simulink model "Full_Car_Model"  (R2020a)
settings: Solver=ode4  StartTime=0  StopTime=3  FixedStep=0.001  RelTol=1e-3
undefined symbols (not defined in the file): a_CG, b_CG, Cs_FL, Cs_FR, Cs_RL, Cs_RR, g, Ip, Ir, Ks_FL, Ks_FR, Ks_RL, Ks_RR, Ms, mus1, mus2, mus3, mus4, tr
settings Model: Creator=anish  LastModifiedBy=anish
settings DataIOCC: ReturnWorkspaceOutputs=off
settings DebuggingCC: PregeneratedLibrarySubsystemCodeDiagnostic=none  ArithmeticOperatorsInVariantConditions=warning
settings SFSimCC: SimUseLocalCustomCode=off  CustomCodeUndefinedFunction=UseInterfaceOnly
settings RTWCC: RTWUseLocalCustomCode=off

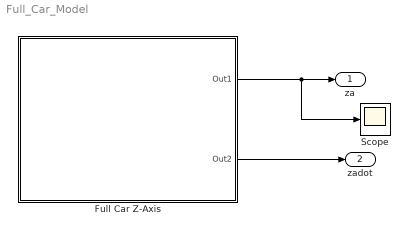
== system Full_Car_Model ==
  Full Car Z-Axis : Subsystem
  Scope : Scope
  za : Outport  VectorParamsAs1DForOutWhenUnconnected=off
  zadot : Outport  Port=2  VectorParamsAs1DForOutWhenUnconnected=off
  wires:
  Full Car Z-Axis/1(Out1) -> Scope/1, za/1
  Full Car Z-Axis/2(Out2) -> zadot/1

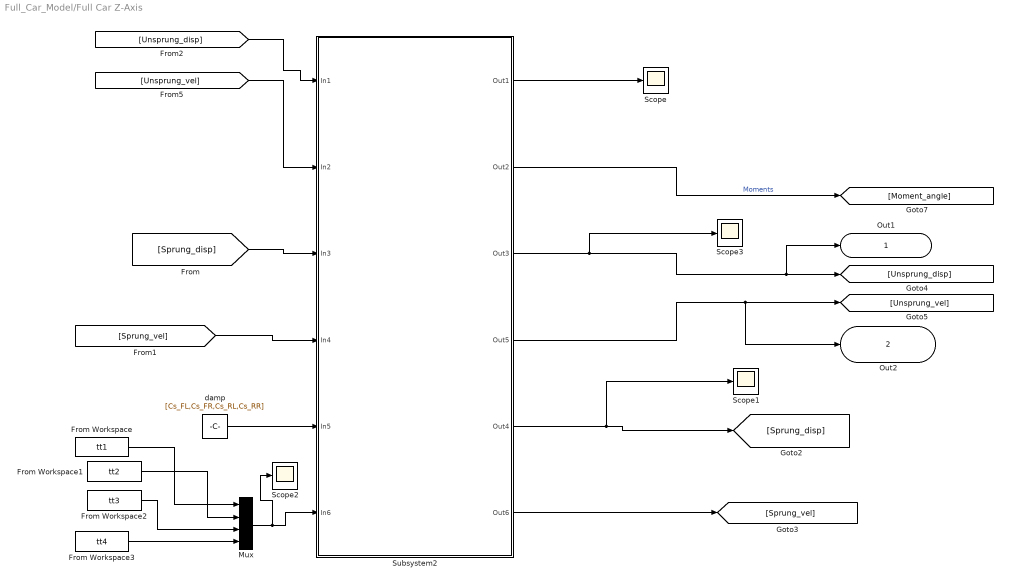
== system Full_Car_Model/Full Car Z-Axis ==
  From Workspace : FromWorkspace  VariableName=tt1  OutputAfterFinalValue=Setting to zero
  From Workspace1 : FromWorkspace  VariableName=tt2  OutputAfterFinalValue=Setting to zero
  From Workspace2 : FromWorkspace  VariableName=tt3  OutputAfterFinalValue=Setting to zero
  From Workspace3 : FromWorkspace  VariableName=tt4  OutputAfterFinalValue=Setting to zero
  Mux : Mux
  Scope{,1..3} (4 alike) : Scope
  Subsystem2 : Subsystem
  damp : Constant  Value=[Cs_FL,Cs_FR,Cs_RL,Cs_RR]
  Out1 : Outport  VectorParamsAs1DForOutWhenUnconnected=off
  Out2 : Outport  Port=2  VectorParamsAs1DForOutWhenUnconnected=off
  wires:
  [Unsprung_disp] -> Subsystem2/1(In1)
  [Unsprung_vel] -> Subsystem2/2(In2)
  damp/1 -> Subsystem2/5(In5)
  [Sprung_disp] -> Subsystem2/3(In3)
  [Sprung_vel] -> Subsystem2/4(In4)
  Subsystem2/3(Out3) -> Scope3/1, Out1/1, [Unsprung_disp]
  Subsystem2/4(Out5) -> Out2/1, [Unsprung_vel]
  Subsystem2/6(Out6) -> [Sprung_vel]
  Subsystem2/2(Out2) -> [Moment_angle]  "Moments"
  Subsystem2/1(Out1) -> Scope/1
  Mux/1 -> Scope2/1, Subsystem2/6(In6)
  From Workspace/1 -> Mux/1
  From Workspace1/1 -> Mux/2
  From Workspace2/1 -> Mux/3
  From Workspace3/1 -> Mux/4
  Subsystem2/5(Out4) -> Scope1/1, [Sprung_disp]

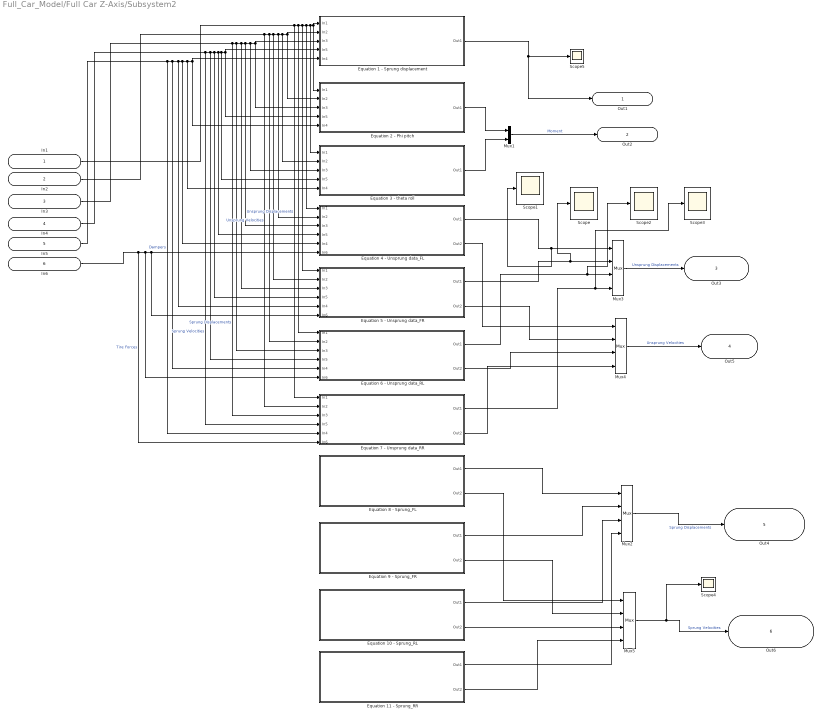
== system Full_Car_Model/Full Car Z-Axis/Subsystem2 ==
  In1 : Inport
  In2 : Inport  Port=2
  In3 : Inport  Port=3
  In4 : Inport  Port=4
  In5 : Inport  Port=5
  In6 : Inport  Port=6
  Equation 1 - Sprung displacement : Subsystem
  Equation 10 - Sprung_RL : Subsystem
  Equation 11 - Sprung_RR : Subsystem
  Equation 2 - Phi pitch : Subsystem
  Equation 3 - theta roll : Subsystem
  Equation 4 - Unsprung data_FL : Subsystem
  Equation 5 - Unsprung data_FR : Subsystem
  Equation 6 - Unsprung data_RL : Subsystem
  Equation 7 - Unsprung data_RR : Subsystem
  Equation 8 - Sprung_FL : Subsystem
  Equation 9 - Sprung_FR : Subsystem
  Mux1 : Mux  Inputs=2
  Mux{2..5} (4 alike) : Mux
  Scope{,1..5} (6 alike) : Scope
  Out1 : Outport  VectorParamsAs1DForOutWhenUnconnected=off
  Out2 : Outport  Port=2  VectorParamsAs1DForOutWhenUnconnected=off
  Out3 : Outport  Port=3  VectorParamsAs1DForOutWhenUnconnected=off
  Out5 : Outport  Port=4  VectorParamsAs1DForOutWhenUnconnected=off
  Out4 : Outport  Port=5  VectorParamsAs1DForOutWhenUnconnected=off
  Out6 : Outport  Port=6  VectorParamsAs1DForOutWhenUnconnected=off
  wires:
  Mux1/1 -> Out2/1  "Moment"
  Equation 2 - Phi pitch/1(Out1) -> Mux1/1
  Equation 3 - theta roll/1(Out1) -> Mux1/2
  In1/1 -> Equation 7 - Unsprung data_RR/1(In1), Equation 6 - Unsprung data_RL/1(In1), Equation 5 - Unsprung data_FR/1(In1), Equation 4 - Unsprung data_FL/1(In1), Equation 3 - theta roll/1(In1), Equation 2 - Phi pitch/1(In1), Equation 1 - Sprung displacement/1(In1)  "Unsprung Displacements"
  In2/1 -> Equation 7 - Unsprung data_RR/2(In2), Equation 6 - Unsprung data_RL/2(In2), Equation 5 - Unsprung data_FR/2(In2), Equation 4 - Unsprung data_FL/2(In2), Equation 3 - theta roll/2(In2), Equation 2 - Phi pitch/2(In2), Equation 1 - Sprung displacement/2(In2)  "Unsprung Velocities"
  In3/1 -> Equation 7 - Unsprung data_RR/3(In3), Equation 6 - Unsprung data_RL/3(In3), Equation 5 - Unsprung data_FR/3(In3), Equation 4 - Unsprung data_FL/3(In3), Equation 3 - theta roll/3(In3), Equation 2 - Phi pitch/3(In3), Equation 1 - Sprung displacement/3(In3)  "Sprung Displacements"
  In4/1 -> Equation 7 - Unsprung data_RR/4(In5), Equation 6 - Unsprung data_RL/4(In5), Equation 5 - Unsprung data_FR/4(In5), Equation 4 - Unsprung data_FL/4(In5), Equation 3 - theta roll/4(In5), Equation 2 - Phi pitch/4(In5), Equation 1 - Sprung displacement/4(In5)  "Sprung Velocities"
  In5/1 -> Equation 7 - Unsprung data_RR/5(In4), Equation 6 - Unsprung data_RL/5(In4), Equation 5 - Unsprung data_FR/5(In4), Equation 4 - Unsprung data_FL/5(In4), Equation 3 - theta roll/5(In4), Equation 2 - Phi pitch/5(In4), Equation 1 - Sprung displacement/5(In4)  "Dampers"
  In6/1 -> Equation 7 - Unsprung data_RR/6(In6), Equation 6 - Unsprung data_RL/6(In6), Equation 5 - Unsprung data_FR/6(In6), Equation 4 - Unsprung data_FL/6(In6)  "Tire Forces"
  Equation 1 - Sprung displacement/1(Out1) -> Out1/1, Scope5/1
  Mux3/1 -> Out3/1  "Unsprung Displacements"
  Mux4/1 -> Out5/1  "Unsprung Velocities"
  Equation 4 - Unsprung data_FL/1(Out1) -> Scope1/1, Mux3/1
  Equation 5 - Unsprung data_FR/1(Out1) -> Scope/1, Mux3/2
  Equation 6 - Unsprung data_RL/1(Out1) -> Scope2/1, Mux3/3
  Equation 7 - Unsprung data_RR/1(Out1) -> Scope3/1, Mux3/4
  Equation 4 - Unsprung data_FL/2(Out2) -> Mux4/1
  Equation 5 - Unsprung data_FR/2(Out2) -> Mux4/2
  Equation 6 - Unsprung data_RL/2(Out2) -> Mux4/3
  Equation 7 - Unsprung data_RR/2(Out2) -> Mux4/4
  Mux2/1 -> Out4/1  "Sprung Displacements"
  Mux5/1 -> Scope4/1, Out6/1  "Sprung Velocities"
  Equation 8 - Sprung_FL/1(Out1) -> Mux2/1
  Equation 9 - Sprung_FR/1(Out1) -> Mux2/2
  Equation 10 - Sprung_RL/1(Out1) -> Mux2/3
  Equation 11 - Sprung_RR/1(Out1) -> Mux2/4
  Equation 8 - Sprung_FL/2(Out2) -> Mux5/1
  Equation 9 - Sprung_FR/2(Out2) -> Mux5/2
  Equation 10 - Sprung_RL/2(Out2) -> Mux5/3
  Equation 11 - Sprung_RR/2(Out2) -> Mux5/4

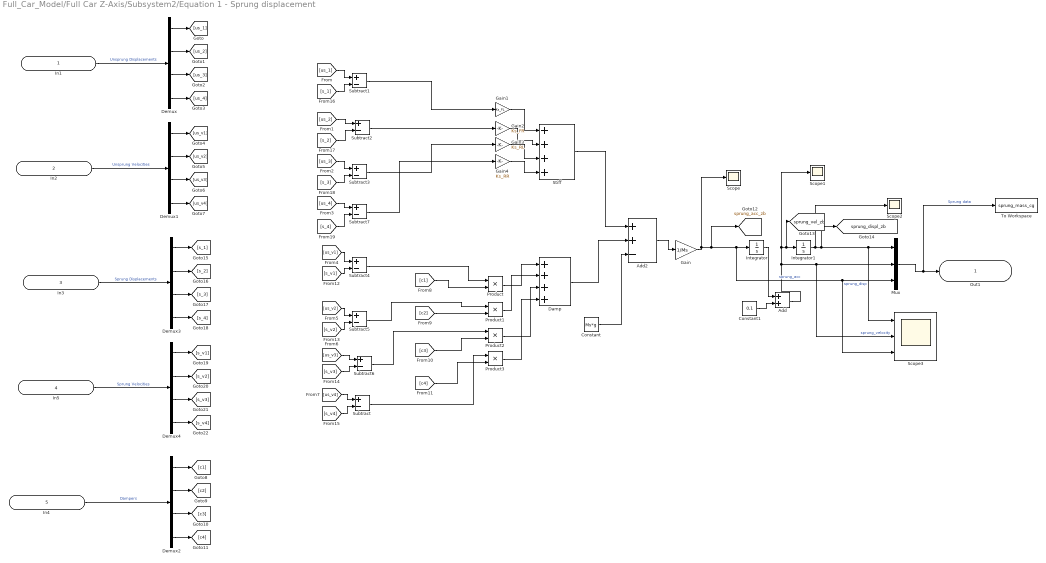
== system Full_Car_Model/Full Car Z-Axis/Subsystem2/Equation 1 - Sprung displacement ==
  In1 : Inport
  In2 : Inport  Port=2
  In3 : Inport  Port=3
  In5 : Inport  Port=4
  In4 : Inport  Port=5
  Add : Sum
  Add2 : Sum  Inputs=++-
  Constant : Constant  Value=Ms*g
  Constant1 : Constant  Value=0.1
  Damp : Sum  Inputs=++++
  Demux{,1..4} (5 alike) : Demux
  Gain : Gain  Gain=1/Ms
  Gain1 : Gain  Gain=Ks_FL
  Gain2 : Gain  Gain=Ks_FR
  Gain3 : Gain  Gain=Ks_RL
  Gain4 : Gain  Gain=Ks_RR
  Integrator : Integrator
  Integrator1 : Integrator  InitialCondition=-0.0177
  Mux : Mux  Inputs=3
  Product{,1..3} (4 alike) : Product
  Scope : Scope
  Scope1 : Scope
  Scope2 : Scope
  Scope3 : Scope  NumInputPorts=3
  Stiff : Sum  Inputs=++++
  Subtract{,1..7} (8 alike) : Sum  Inputs=+-
  To Workspace : ToWorkspace  VariableName=sprung_mass_cg  SampleTime=-1
      settings: Save2DSignal=2-D array (concatenate along first dimension)
  Out1 : Outport  VectorParamsAs1DForOutWhenUnconnected=off
  tag scope: sprung_acc_zb=global, sprung_displ_zb=global, sprung_vel_zb=global
  wires:
  In1/1 -> Demux/1  "Unsprung Displacements"
  Add2/1 -> Gain/1
  Damp/1 -> Add2/2
  Constant/1 -> Add2/3
  Gain/1 -> Scope/1, [sprung_acc_zb], Scope3/3, Mux/3, Integrator/1  "sprung_acc"
  Mux/1 -> To Workspace/1, Out1/1  "Sprung data"
  Demux/1 -> [us_1]
  Demux/2 -> [us_2]
  Demux/3 -> [us_3]
  Demux/4 -> [us_4]
  In2/1 -> Demux1/1  "Unsprung Velocities"
  Demux1/1 -> [us_v1]
  Demux1/4 -> [us_v4]
  Demux1/2 -> [us_v2]
  Demux1/3 -> [us_v3]
  In4/1 -> Demux2/1  "Dampers"
  Demux2/3 -> [c3]
  Demux2/2 -> [c2]
  Demux2/4 -> [c4]
  Demux2/1 -> [c1]
  Integrator1/1 -> Scope2/1, [sprung_displ_zb], Scope3/1, Mux/1  "sprung_disp"
  Gain1/1 -> Stiff/1
  Gain2/1 -> Stiff/2
  Gain3/1 -> Stiff/3
  Gain4/1 -> Stiff/4
  [c1] -> Product/2
  [c4] -> Product3/2
  [c3] -> Product2/2
  [c2] -> Product1/2
  Product/1 -> Damp/1
  Product1/1 -> Damp/2
  Product2/1 -> Damp/3
  Product3/1 -> Damp/4
  Demux4/4 -> [s_v4]
  Demux3/2 -> [s_2]
  Demux4/1 -> [s_v1]
  Demux3/4 -> [s_4]
  Demux3/3 -> [s_3]
  Demux3/1 -> [s_1]
  Demux4/2 -> [s_v2]
  Demux4/3 -> [s_v3]
  In5/1 -> Demux4/1  "Sprung Velocities"
  In3/1 -> Demux3/1  "Sprung Displacements"
  [us_v1] -> Subtract4/1
  [s_v1] -> Subtract4/2
  [us_v2] -> Subtract5/1
  [s_v2] -> Subtract5/2
  [us_v3] -> Subtract6/1
  [s_v3] -> Subtract6/2
  [us_v4] -> Subtract/1
  [s_v4] -> Subtract/2
  Subtract4/1 -> Product/1
  Subtract5/1 -> Product1/1
  Subtract6/1 -> Product2/1
  Subtract/1 -> Product3/1
  [us_1] -> Subtract1/1
  [s_1] -> Subtract1/2
  [us_2] -> Subtract2/1
  [s_2] -> Subtract2/2
  [us_3] -> Subtract3/1
  [s_3] -> Subtract3/2
  [us_4] -> Subtract7/1
  [s_4] -> Subtract7/2
  Stiff/1 -> Add2/1
  Subtract1/1 -> Gain1/1
  Subtract2/1 -> Gain2/1
  Subtract3/1 -> Gain3/1
  Subtract7/1 -> Gain4/1
  Constant1/1 -> Add/2
  Integrator/1 -> Add/1
  Add/1 -> Scope3/2, Mux/2, Scope1/1, [sprung_vel_zb], Integrator1/1  "sprung_velocity"

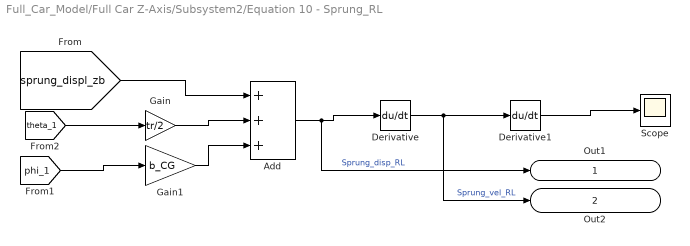
== system Full_Car_Model/Full Car Z-Axis/Subsystem2/Equation 10 - Sprung_RL ==
  Add : Sum  Inputs=+++
  Derivative : Derivative
  Derivative1 : Derivative
  Gain : Gain  Gain=tr/2
  Gain1 : Gain  Gain=b_CG
  Scope : Scope
  Out1 : Outport  VectorParamsAs1DForOutWhenUnconnected=off
  Out2 : Outport  Port=2  VectorParamsAs1DForOutWhenUnconnected=off
  wires:
  [sprung_displ_zb] -> Add/1
  Gain/1 -> Add/2
  Gain1/1 -> Add/3
  [phi_1] -> Gain1/1
  [theta_1] -> Gain/1
  Add/1 -> Out1/1, Derivative/1  "Sprung_disp_RL"
  Derivative/1 -> Out2/1, Derivative1/1  "Sprung_vel_RL"
  Derivative1/1 -> Scope/1

== system Full_Car_Model/Full Car Z-Axis/Subsystem2/Equation 11 - Sprung_RR ==
  Add : Sum  Inputs=+-+
  Derivative : Derivative
  Derivative1 : Derivative
  Gain : Gain  Gain=tr/2
  Gain1 : Gain  Gain=b_CG
  Scope : Scope
  Out1 : Outport  VectorParamsAs1DForOutWhenUnconnected=off
  Out2 : Outport  Port=2  VectorParamsAs1DForOutWhenUnconnected=off
  wires:
  [sprung_displ_zb] -> Add/1
  Gain/1 -> Add/2
  Gain1/1 -> Add/3
  [phi_1] -> Gain1/1
  [theta_1] -> Gain/1
  Add/1 -> Out1/1, Derivative/1  "Sprung_disp_RR"
  Derivative/1 -> Out2/1, Derivative1/1  "Sprung_vel_RR"
  Derivative1/1 -> Scope/1

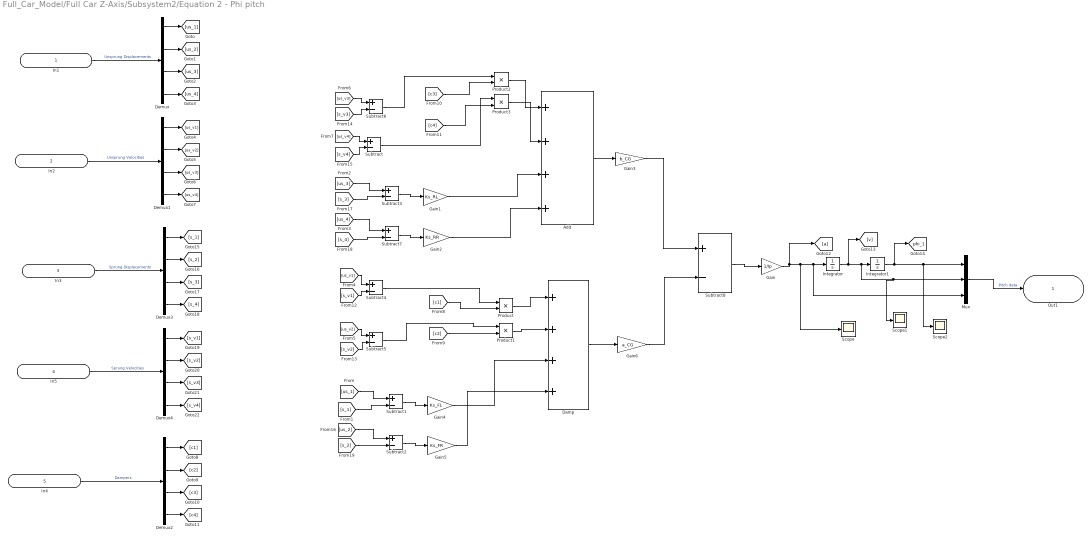
== system Full_Car_Model/Full Car Z-Axis/Subsystem2/Equation 2 - Phi pitch ==
  In1 : Inport
  In2 : Inport  Port=2
  In3 : Inport  Port=3
  In5 : Inport  Port=4
  In4 : Inport  Port=5
  Add : Sum  Inputs=++++
  Damp : Sum  Inputs=++++
  Demux{,1..4} (5 alike) : Demux
  Gain : Gain  Gain=1/Ip
  Gain1 : Gain  Gain=Ks_RL
  Gain2 : Gain  Gain=Ks_RR
  Gain3 : Gain  Gain=b_CG
  Gain4 : Gain  Gain=Ks_FL
  Gain5 : Gain  Gain=Ks_FR
  Gain6 : Gain  Gain=a_CG
  Integrator : Integrator  UpperSaturationLimit=0.00001  LowerSaturationLimit=-0.00001
  Integrator1 : Integrator  UpperSaturationLimit=0.00001  LowerSaturationLimit=-0.00001
  Mux : Mux  Inputs=3
  Product{,1..3} (4 alike) : Product
  Scope : Scope
  Scope1 : Scope
  Scope2 : Scope
  Subtract{,1..8} (9 alike) : Sum  Inputs=+-
  Out1 : Outport  VectorParamsAs1DForOutWhenUnconnected=off
  tag scope: phi_1=global
  wires:
  In1/1 -> Demux/1  "Unsprung Displacements"
  Subtract8/1 -> Gain/1
  Gain/1 -> [a], Scope/1, Mux/3, Integrator/1
  Integrator/1 -> [v], Scope1/1, Mux/2, Integrator1/1
  Mux/1 -> Out1/1  "Pitch data"
  Demux/1 -> [us_1]
  Demux/2 -> [us_2]
  Demux/3 -> [us_3]
  Demux/4 -> [us_4]
  In2/1 -> Demux1/1  "Unsprung Velocities"
  Demux1/1 -> [us_v1]
  Demux1/4 -> [us_v4]
  Demux1/2 -> [us_v2]
  Demux1/3 -> [us_v3]
  In4/1 -> Demux2/1  "Dampers"
  Demux2/3 -> [c3]
  Demux2/2 -> [c2]
  Demux2/4 -> [c4]
  Demux2/1 -> [c1]
  Integrator1/1 -> [phi_1], Scope2/1, Mux/1
  [c1] -> Product/2
  [c2] -> Product1/2
  Product/1 -> Damp/1
  Product1/1 -> Damp/2
  Demux4/4 -> [s_v4]
  Demux3/2 -> [s_2]
  Demux4/1 -> [s_v1]
  Demux3/4 -> [s_4]
  Demux3/3 -> [s_3]
  Demux3/1 -> [s_1]
  Demux4/2 -> [s_v2]
  Demux4/3 -> [s_v3]
  In5/1 -> Demux4/1  "Sprung Velocities"
  In3/1 -> Demux3/1  "Sprung Displacements"
  [us_v1] -> Subtract4/1
  [s_v1] -> Subtract4/2
  [us_v2] -> Subtract5/1
  [s_v2] -> Subtract5/2
  Subtract4/1 -> Product/1
  Subtract5/1 -> Product1/1
  [us_2] -> Subtract2/1
  [s_1] -> Subtract1/2
  Subtract2/1 -> Gain5/1
  Subtract1/1 -> Gain4/1
  [us_1] -> Subtract1/1
  [s_2] -> Subtract2/2
  Gain4/1 -> Damp/3
  Gain5/1 -> Damp/4
  Damp/1 -> Gain6/1
  Product2/1 -> Add/1
  Subtract3/1 -> Gain1/1
  Gain1/1 -> Add/3
  [c3] -> Product2/2
  [c4] -> Product3/2
  [s_v3] -> Subtract6/2
  [us_v4] -> Subtract/1
  Subtract6/1 -> Product2/1
  Subtract/1 -> Product3/1
  [s_3] -> Subtract3/2
  Gain2/1 -> Add/4
  [s_v4] -> Subtract/2
  [us_v3] -> Subtract6/1
  Subtract7/1 -> Gain2/1
  Product3/1 -> Add/2
  [us_3] -> Subtract3/1
  [s_4] -> Subtract7/2
  Add/1 -> Gain3/1
  [us_4] -> Subtract7/1
  Gain3/1 -> Subtract8/1
  Gain6/1 -> Subtract8/2

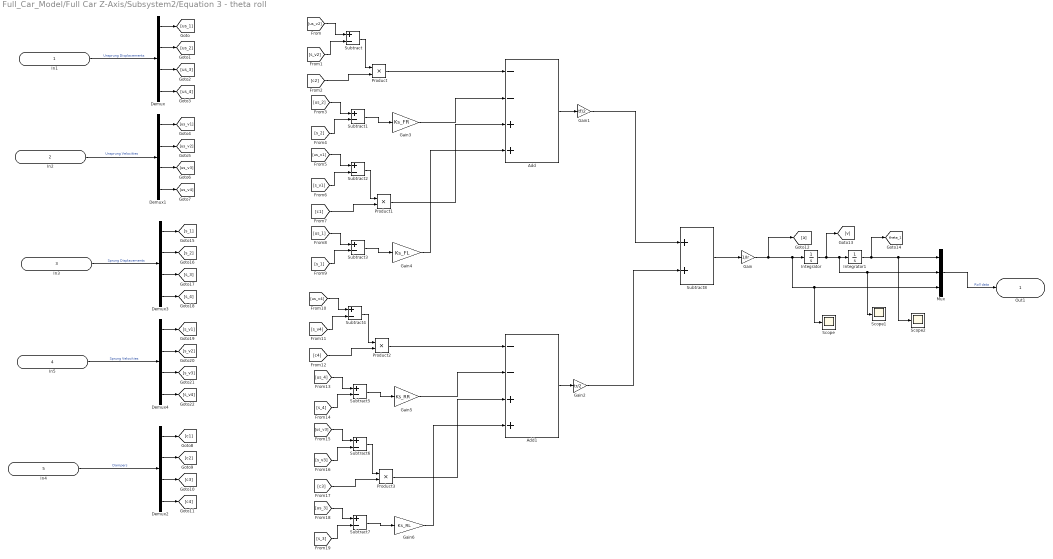
== system Full_Car_Model/Full Car Z-Axis/Subsystem2/Equation 3 - theta roll ==
  In1 : Inport
  In2 : Inport  Port=2
  In3 : Inport  Port=3
  In5 : Inport  Port=4
  In4 : Inport  Port=5
  Add : Sum  Inputs=--++
  Add1 : Sum  Inputs=--++
  Demux{,1..4} (5 alike) : Demux
  Gain : Gain  Gain=1/Ir
  Gain1 : Gain  Gain=tf/2
  Gain2 : Gain  Gain=tr/2
  Gain3 : Gain  Gain=Ks_FR
  Gain4 : Gain  Gain=Ks_FL
  Gain5 : Gain  Gain=Ks_RR
  Gain6 : Gain  Gain=Ks_RL
  Integrator : Integrator  UpperSaturationLimit=0.00001  LowerSaturationLimit=-0.00001
  Integrator1 : Integrator  UpperSaturationLimit=0.00001  LowerSaturationLimit=-0.00001
  Mux : Mux  Inputs=3
  Product{,1..3} (4 alike) : Product
  Scope : Scope
  Scope1 : Scope
  Scope2 : Scope
  Subtract{,1..7} (8 alike) : Sum  Inputs=+-
  Subtract8 : Sum
  Out1 : Outport  VectorParamsAs1DForOutWhenUnconnected=off
  tag scope: theta_1=global
  wires:
  In1/1 -> Demux/1  "Unsprung Displacements"
  Subtract8/1 -> Gain/1
  Integrator/1 -> [v], Scope1/1, Mux/2, Integrator1/1
  Mux/1 -> Out1/1  "Roll data"
  Demux/1 -> [us_1]
  Demux/2 -> [us_2]
  Demux/3 -> [us_3]
  Demux/4 -> [us_4]
  In2/1 -> Demux1/1  "Unsprung Velocities"
  Demux1/1 -> [us_v1]
  Demux1/4 -> [us_v4]
  Demux1/2 -> [us_v2]
  Demux1/3 -> [us_v3]
  In4/1 -> Demux2/1  "Dampers"
  Demux2/3 -> [c3]
  Demux2/2 -> [c2]
  Demux2/4 -> [c4]
  Demux2/1 -> [c1]
  Integrator1/1 -> [theta_1], Scope2/1, Mux/1
  Demux4/4 -> [s_v4]
  Demux3/2 -> [s_2]
  Demux4/1 -> [s_v1]
  Demux3/4 -> [s_4]
  Demux3/3 -> [s_3]
  Demux3/1 -> [s_1]
  Demux4/2 -> [s_v2]
  Demux4/3 -> [s_v3]
  In5/1 -> Demux4/1  "Sprung Velocities"
  In3/1 -> Demux3/1  "Sprung Displacements"
  Add/1 -> Gain1/1
  Add1/1 -> Gain2/1
  [us_v2] -> Subtract/1
  [s_v2] -> Subtract/2
  Subtract/1 -> Product/1
  [c2] -> Product/2
  Product/1 -> Add/1
  [s_2] -> Subtract1/2
  [us_2] -> Subtract1/1
  Subtract1/1 -> Gain3/1
  Gain3/1 -> Add/2
  [c1] -> Product1/2
  [s_v1] -> Subtract2/2
  Subtract2/1 -> Product1/1
  [us_v1] -> Subtract2/1
  Product1/1 -> Add/3
  [s_1] -> Subtract3/2
  [us_1] -> Subtract3/1
  Subtract3/1 -> Gain4/1
  Gain4/1 -> Add/4
  [us_v3] -> Subtract6/1
  [c3] -> Product3/2
  [s_v3] -> Subtract6/2
  [s_4] -> Subtract5/2
  [us_4] -> Subtract5/1
  [s_3] -> Subtract7/2
  Subtract5/1 -> Gain5/1
  Product3/1 -> Add1/3
  Product2/1 -> Add1/1
  Gain5/1 -> Add1/2
  Subtract6/1 -> Product3/1
  Gain6/1 -> Add1/4
  [us_3] -> Subtract7/1
  [c4] -> Product2/2
  [s_v4] -> Subtract4/2
  Subtract7/1 -> Gain6/1
  Subtract4/1 -> Product2/1
  [us_v4] -> Subtract4/1
  Gain1/1 -> Subtract8/1
  Gain2/1 -> Subtract8/2
  Gain/1 -> [a], Scope/1, Mux/3, Integrator/1

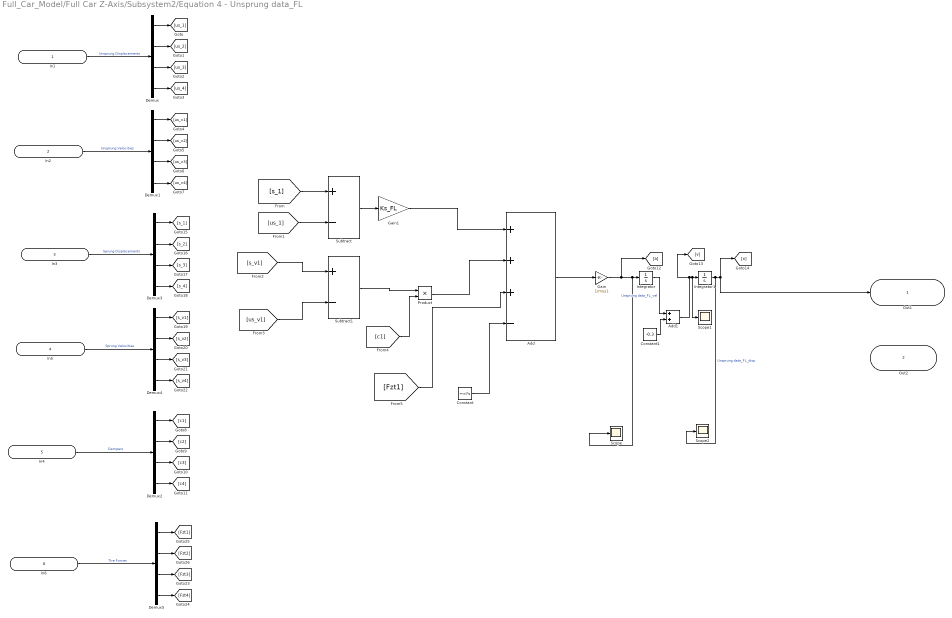
== system Full_Car_Model/Full Car Z-Axis/Subsystem2/Equation 4 - Unsprung data_FL ==
  In1 : Inport
  In2 : Inport  Port=2
  In3 : Inport  Port=3
  In5 : Inport  Port=4
  In4 : Inport  Port=5
  In6 : Inport  Port=6
  Add : Sum  Inputs=+++-
  Add1 : Sum
  Constant : Constant  Value=mus1*g
  Constant1 : Constant  Value=-0.3
  Demux{,1..5} (6 alike) : Demux
  Gain : Gain  Gain=1/mus1
  Gain1 : Gain  Gain=Ks_FL
  Integrator : Integrator
  Integrator1 : Integrator  InitialCondition=-0.0177
  Product : Product
  Scope : Scope
  Scope1 : Scope
  Scope2 : Scope
  Subtract : Sum  Inputs=+-
  Subtract1 : Sum  Inputs=+-
  Out1 : Outport  VectorParamsAs1DForOutWhenUnconnected=off
  Out2 : Outport  Port=2  VectorParamsAs1DForOutWhenUnconnected=off
  wires:
  In1/1 -> Demux/1  "Unsprung Displacements"
  Add/1 -> Gain/1
  Integrator1/1 -> Scope2/1, Out1/1, [x]  "Unsprung data_FL_disp"
  Demux/1 -> [us_1]
  Demux/2 -> [us_2]
  Demux/3 -> [us_3]
  Demux/4 -> [us_4]
  In2/1 -> Demux1/1  "Unsprung Velocities"
  Demux1/1 -> [us_v1]
  Demux1/4 -> [us_v4]
  Demux1/2 -> [us_v2]
  Demux1/3 -> [us_v3]
  In4/1 -> Demux2/1  "Dampers"
  Demux2/3 -> [c3]
  Demux2/2 -> [c2]
  Demux2/4 -> [c4]
  Demux2/1 -> [c1]
  Demux4/4 -> [s_v4]
  Demux3/2 -> [s_2]
  Demux4/1 -> [s_v1]
  Demux3/4 -> [s_4]
  Demux3/3 -> [s_3]
  Demux3/1 -> [s_1]
  Demux4/2 -> [s_v2]
  Demux4/3 -> [s_v3]
  In5/1 -> Demux4/1  "Sprung Velocities"
  In3/1 -> Demux3/1  "Sprung Displacements"
  In6/1 -> Demux5/1  "Tire Forces"
  Demux5/2 -> [Fzt2]
  Demux5/3 -> [Fzt3]
  Demux5/1 -> [Fzt1]
  Demux5/4 -> [Fzt4]
  [us_1] -> Subtract/2
  [s_1] -> Subtract/1
  Subtract/1 -> Gain1/1
  [s_v1] -> Subtract1/1
  [us_v1] -> Subtract1/2
  Subtract1/1 -> Product/1
  [c1] -> Product/2
  Gain1/1 -> Add/1
  Product/1 -> Add/2
  [Fzt1] -> Add/3
  Constant/1 -> Add/4
  Gain/1 -> [a], Scope/1, Integrator/1
  Constant1/1 -> Add1/2
  Integrator/1 -> Add1/1  "Unsprung data_FL_vel"
  Add1/1 -> Scope1/1, Integrator1/1, [v]

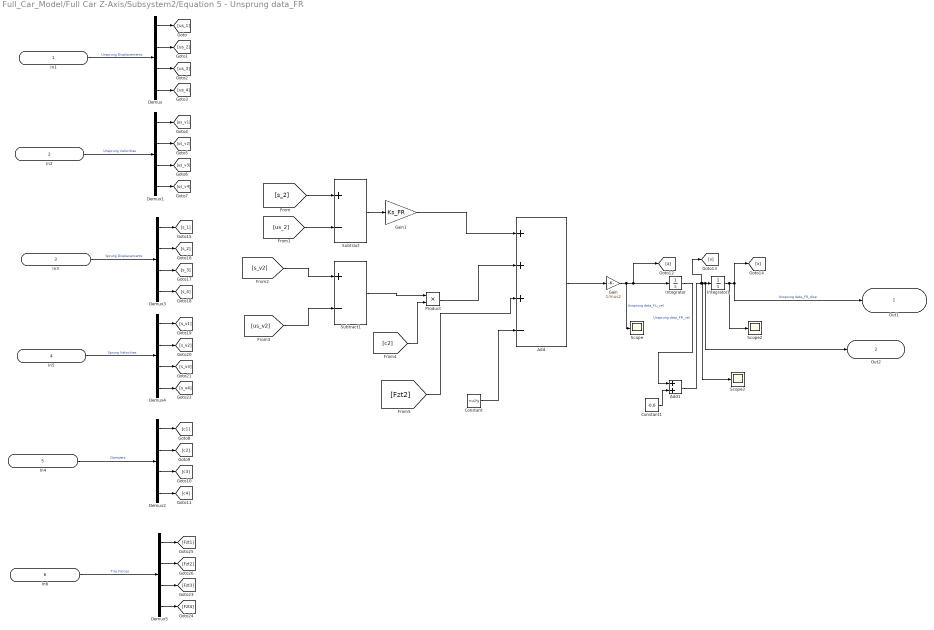
== system Full_Car_Model/Full Car Z-Axis/Subsystem2/Equation 5 - Unsprung data_FR ==
  In1 : Inport
  In2 : Inport  Port=2
  In3 : Inport  Port=3
  In5 : Inport  Port=4
  In4 : Inport  Port=5
  In6 : Inport  Port=6
  Add : Sum  Inputs=+++-
  Add1 : Sum
  Constant : Constant  Value=mus2*g
  Constant1 : Constant  Value=-0.6
  Demux{,1..5} (6 alike) : Demux
  Gain : Gain  Gain=1/mus2
  Gain1 : Gain  Gain=Ks_FR
  Integrator : Integrator
  Integrator1 : Integrator  InitialCondition=-0.0177
  Product : Product
  Scope : Scope
  Scope2 : Scope
  Scope3 : Scope
  Subtract : Sum  Inputs=+-
  Subtract1 : Sum  Inputs=+-
  Out1 : Outport  VectorParamsAs1DForOutWhenUnconnected=off
  Out2 : Outport  Port=2  VectorParamsAs1DForOutWhenUnconnected=off
  wires:
  In1/1 -> Demux/1  "Unsprung Displacements"
  Add/1 -> Gain/1
  Integrator1/1 -> Scope2/1, Out1/1, [x]  "Unsprung data_FR_disp"
  Demux/1 -> [us_1]
  Demux/2 -> [us_2]
  Demux/3 -> [us_3]
  Demux/4 -> [us_4]
  In2/1 -> Demux1/1  "Unsprung Velocities"
  Demux1/1 -> [us_v1]
  Demux1/4 -> [us_v4]
  Demux1/2 -> [us_v2]
  Demux1/3 -> [us_v3]
  In4/1 -> Demux2/1  "Dampers"
  Demux2/3 -> [c3]
  Demux2/2 -> [c2]
  Demux2/4 -> [c4]
  Demux2/1 -> [c1]
  Demux4/4 -> [s_v4]
  Demux3/2 -> [s_2]
  Demux4/1 -> [s_v1]
  Demux3/4 -> [s_4]
  Demux3/3 -> [s_3]
  Demux3/1 -> [s_1]
  Demux4/2 -> [s_v2]
  Demux4/3 -> [s_v3]
  In5/1 -> Demux4/1  "Sprung Velocities"
  In3/1 -> Demux3/1  "Sprung Displacements"
  In6/1 -> Demux5/1  "Tire Forces"
  Demux5/2 -> [Fzt2]
  Demux5/3 -> [Fzt3]
  Demux5/1 -> [Fzt1]
  Demux5/4 -> [Fzt4]
  [us_2] -> Subtract/2
  [s_2] -> Subtract/1
  Subtract/1 -> Gain1/1
  [s_v2] -> Subtract1/1
  [us_v2] -> Subtract1/2
  Subtract1/1 -> Product/1
  [c2] -> Product/2
  Gain1/1 -> Add/1
  Product/1 -> Add/2
  [Fzt2] -> Add/3
  Constant/1 -> Add/4
  Constant1/1 -> Add1/2
  Gain/1 -> Scope/1, [a], Integrator/1  "Unsprung data_FL_vel"
  Integrator/1 -> Add1/1  "Unsprung data_FR_vel"
  Add1/1 -> [v], Scope3/1, Out2/1, Integrator1/1

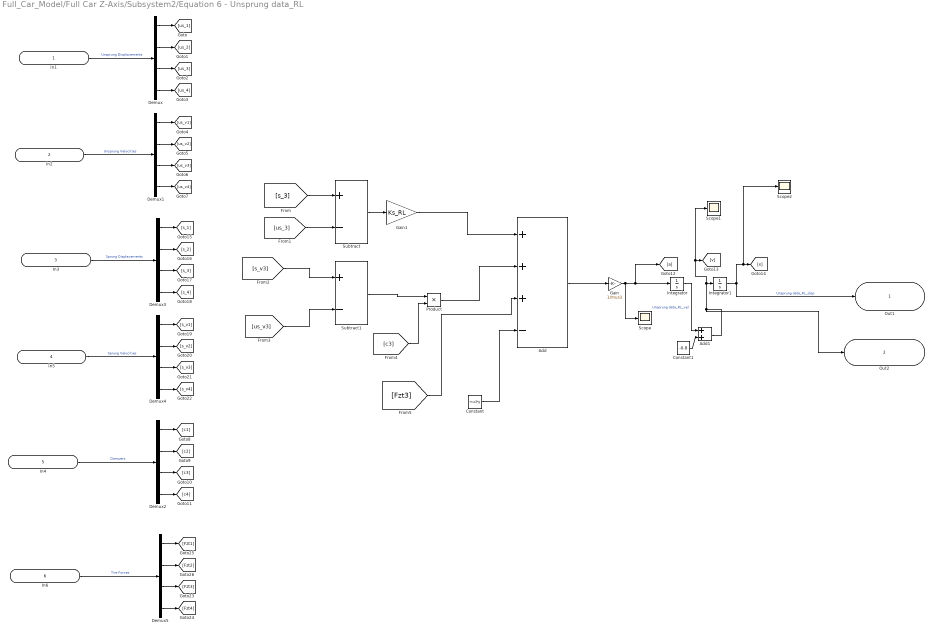
== system Full_Car_Model/Full Car Z-Axis/Subsystem2/Equation 6 - Unsprung data_RL ==
  In1 : Inport
  In2 : Inport  Port=2
  In3 : Inport  Port=3
  In5 : Inport  Port=4
  In4 : Inport  Port=5
  In6 : Inport  Port=6
  Add : Sum  Inputs=+++-
  Add1 : Sum
  Constant : Constant  Value=mus3*g
  Constant1 : Constant  Value=-0.8
  Demux{,1..5} (6 alike) : Demux
  Gain : Gain  Gain=1/mus3
  Gain1 : Gain  Gain=Ks_RL
  Integrator : Integrator
  Integrator1 : Integrator  InitialCondition=-0.0177
  Product : Product
  Scope : Scope
  Scope1 : Scope
  Scope2 : Scope
  Subtract : Sum  Inputs=+-
  Subtract1 : Sum  Inputs=+-
  Out1 : Outport  VectorParamsAs1DForOutWhenUnconnected=off
  Out2 : Outport  Port=2  VectorParamsAs1DForOutWhenUnconnected=off
  wires:
  In1/1 -> Demux/1  "Unsprung Displacements"
  Add/1 -> Gain/1
  Gain/1 -> Scope/1, [a], Integrator/1
  Integrator1/1 -> Out1/1, Scope2/1, [x]  "Unsprung data_RL_disp"
  Demux/1 -> [us_1]
  Demux/2 -> [us_2]
  Demux/3 -> [us_3]
  Demux/4 -> [us_4]
  In2/1 -> Demux1/1  "Unsprung Velocities"
  Demux1/1 -> [us_v1]
  Demux1/4 -> [us_v4]
  Demux1/2 -> [us_v2]
  Demux1/3 -> [us_v3]
  In4/1 -> Demux2/1  "Dampers"
  Demux2/3 -> [c3]
  Demux2/2 -> [c2]
  Demux2/4 -> [c4]
  Demux2/1 -> [c1]
  Demux4/4 -> [s_v4]
  Demux3/2 -> [s_2]
  Demux4/1 -> [s_v1]
  Demux3/4 -> [s_4]
  Demux3/3 -> [s_3]
  Demux3/1 -> [s_1]
  Demux4/2 -> [s_v2]
  Demux4/3 -> [s_v3]
  In5/1 -> Demux4/1  "Sprung Velocities"
  In3/1 -> Demux3/1  "Sprung Displacements"
  In6/1 -> Demux5/1  "Tire Forces"
  Demux5/2 -> [Fzt2]
  Demux5/3 -> [Fzt3]
  Demux5/1 -> [Fzt1]
  Demux5/4 -> [Fzt4]
  [us_3] -> Subtract/2
  [s_3] -> Subtract/1
  Subtract/1 -> Gain1/1
  [s_v3] -> Subtract1/1
  [us_v3] -> Subtract1/2
  Subtract1/1 -> Product/1
  [c3] -> Product/2
  Gain1/1 -> Add/1
  Product/1 -> Add/2
  [Fzt3] -> Add/3
  Constant/1 -> Add/4
  Constant1/1 -> Add1/2
  Integrator/1 -> Add1/1  "Unsprung data_RL_vel"
  Add1/1 -> Scope1/1, [v], Integrator1/1, Out2/1

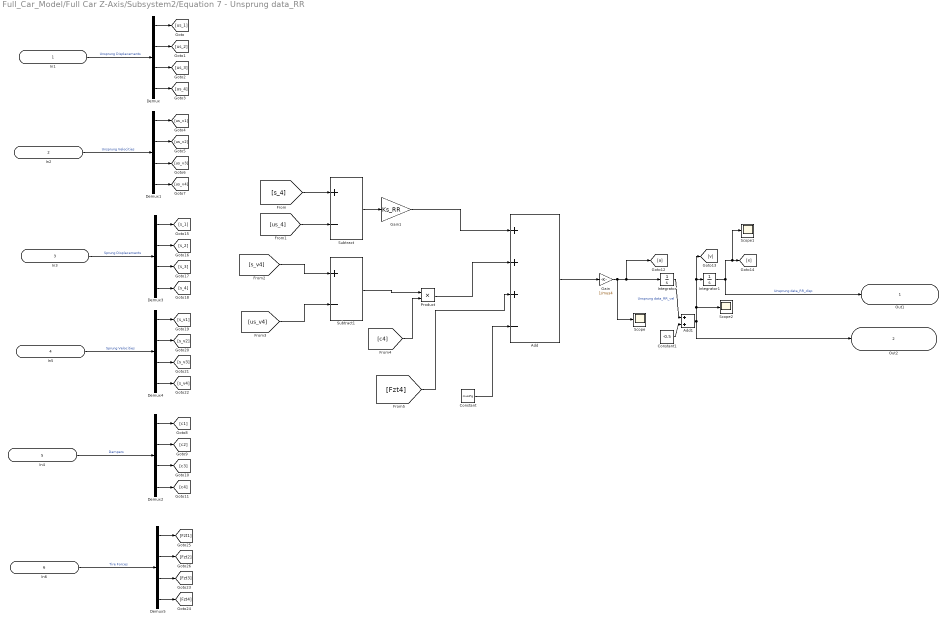
== system Full_Car_Model/Full Car Z-Axis/Subsystem2/Equation 7 - Unsprung data_RR ==
  In1 : Inport
  In2 : Inport  Port=2
  In3 : Inport  Port=3
  In5 : Inport  Port=4
  In4 : Inport  Port=5
  In6 : Inport  Port=6
  Add : Sum  Inputs=+++-
  Add1 : Sum
  Constant : Constant  Value=mus4*g
  Constant1 : Constant  Value=-0.5
  Demux{,1..5} (6 alike) : Demux
  Gain : Gain  Gain=1/mus4
  Gain1 : Gain  Gain=Ks_RR
  Integrator : Integrator
  Integrator1 : Integrator  InitialCondition=-0.0177
  Product : Product
  Scope : Scope
  Scope1 : Scope
  Scope2 : Scope
  Subtract : Sum  Inputs=+-
  Subtract1 : Sum  Inputs=+-
  Out1 : Outport  VectorParamsAs1DForOutWhenUnconnected=off
  Out2 : Outport  Port=2  VectorParamsAs1DForOutWhenUnconnected=off
  wires:
  In1/1 -> Demux/1  "Unsprung Displacements"
  Add/1 -> Gain/1
  Gain/1 -> Scope/1, [a], Integrator/1
  Integrator1/1 -> Out1/1, Scope1/1, [x]  "Unsprung data_RR_disp"
  Demux/1 -> [us_1]
  Demux/2 -> [us_2]
  Demux/3 -> [us_3]
  Demux/4 -> [us_4]
  In2/1 -> Demux1/1  "Unsprung Velocities"
  Demux1/1 -> [us_v1]
  Demux1/4 -> [us_v4]
  Demux1/2 -> [us_v2]
  Demux1/3 -> [us_v3]
  In4/1 -> Demux2/1  "Dampers"
  Demux2/3 -> [c3]
  Demux2/2 -> [c2]
  Demux2/4 -> [c4]
  Demux2/1 -> [c1]
  Demux4/4 -> [s_v4]
  Demux3/2 -> [s_2]
  Demux4/1 -> [s_v1]
  Demux3/4 -> [s_4]
  Demux3/3 -> [s_3]
  Demux3/1 -> [s_1]
  Demux4/2 -> [s_v2]
  Demux4/3 -> [s_v3]
  In5/1 -> Demux4/1  "Sprung Velocities"
  In3/1 -> Demux3/1  "Sprung Displacements"
  In6/1 -> Demux5/1  "Tire Forces"
  Demux5/2 -> [Fzt2]
  Demux5/3 -> [Fzt3]
  Demux5/1 -> [Fzt1]
  Demux5/4 -> [Fzt4]
  [us_4] -> Subtract/2
  [s_4] -> Subtract/1
  Subtract/1 -> Gain1/1
  [s_v4] -> Subtract1/1
  [us_v4] -> Subtract1/2
  Subtract1/1 -> Product/1
  [c4] -> Product/2
  Gain1/1 -> Add/1
  Product/1 -> Add/2
  [Fzt4] -> Add/3
  Constant/1 -> Add/4
  Constant1/1 -> Add1/2
  Integrator/1 -> Add1/1  "Unsprung data_RR_vel"
  Add1/1 -> [v], Integrator1/1, Scope2/1, Out2/1

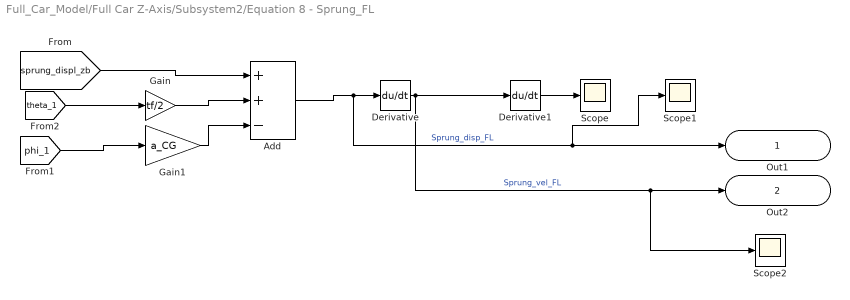
== system Full_Car_Model/Full Car Z-Axis/Subsystem2/Equation 8 - Sprung_FL ==
  Add : Sum  Inputs=++-
  Derivative : Derivative
  Derivative1 : Derivative
  Gain : Gain  Gain=tf/2
  Gain1 : Gain  Gain=a_CG
  Scope : Scope
  Scope1 : Scope
  Scope2 : Scope
  Out1 : Outport  VectorParamsAs1DForOutWhenUnconnected=off
  Out2 : Outport  Port=2  VectorParamsAs1DForOutWhenUnconnected=off
  wires:
  [sprung_displ_zb] -> Add/1
  Gain/1 -> Add/2
  Gain1/1 -> Add/3
  [phi_1] -> Gain1/1
  [theta_1] -> Gain/1
  Add/1 -> Scope1/1, Out1/1, Derivative/1  "Sprung_disp_FL"
  Derivative/1 -> Scope2/1, Out2/1, Derivative1/1  "Sprung_vel_FL"
  Derivative1/1 -> Scope/1

== system Full_Car_Model/Full Car Z-Axis/Subsystem2/Equation 9 - Sprung_FR ==
  Add : Sum  Inputs=+--
  Derivative : Derivative
  Derivative1 : Derivative
  Gain : Gain  Gain=tf/2
  Gain1 : Gain  Gain=a_CG
  Scope : Scope
  Out1 : Outport  VectorParamsAs1DForOutWhenUnconnected=off
  Out2 : Outport  Port=2  VectorParamsAs1DForOutWhenUnconnected=off
  wires:
  [sprung_displ_zb] -> Add/1
  Gain/1 -> Add/2
  Gain1/1 -> Add/3
  [phi_1] -> Gain1/1
  [theta_1] -> Gain/1
  Add/1 -> Out1/1, Derivative/1  "Sprung_disp_FR"
  Derivative/1 -> Out2/1, Derivative1/1  "Sprung_vel_FL"
  Derivative1/1 -> Scope/1
